simulink model "OT_Test"  (Simulink 8.1)
settings: Solver=ode45  StartTime=0.0  StopTime=100  RelTol=1e-3
values from neighbouring files (symbols this model uses):
  KD1 = x(3)    [FA_FACTS.m]
  KI1 = x(2)    [FA_FACTS.m]
  KP1 = x(1)    [FA_FACTS.m]
  N1 = x(4)    [FA_FACTS.m]
libraries: simulink x1
settings Model: Creator=RS Debdeep Saha  LastModifiedBy=RS Debdeep Saha
settings SolverCC: ZeroCrossControl=DisableAll
settings DataIOCC: SignalLoggingSaveFormat=Dataset
settings OptimizationCC: ExpressionDepthLimit=128
settings DebuggingCC: FcnCallInpInsideContextMsg=EnableAllAsError
settings GRTTargetCC: CombineOutputUpdateFcns=on  GRTInterface=off

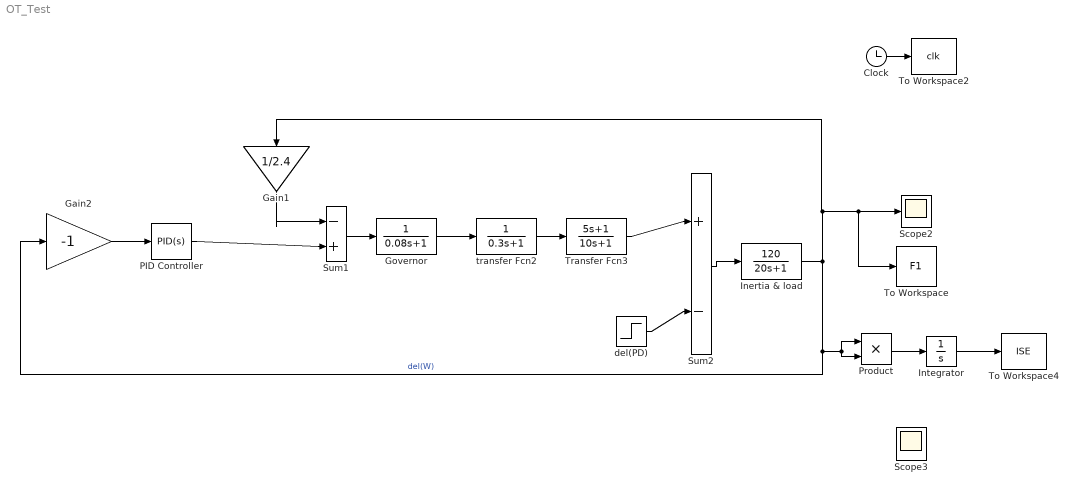
== system OT_Test ==
  Clock : Clock
  Gain1 : Gain  Gain=1/2.4
  Gain2 : Gain  Gain=-1
  Governor : TransferFcn  Denominator=[0.08 1]
  Inertia & load : TransferFcn  Numerator=[120]  Denominator=[20 1]
  Integrator : Integrator
  PID Controller : simulink/Continuous/PID Controller  Controller=PID  TimeDomain=Continuous-time  SampleTime=1  IntegratorMethod=Forward Euler  FilterMethod=Forward Euler  Form=Parallel  P=KP1  I=KI1  D=KD1  N=N1  InitialConditionSource=internal  InitialConditionForIntegrator=0  InitialConditionForFilter=0  ExternalReset=none  LimitOutput=off  UpperSaturationLimit=inf  LowerSaturationLimit=-inf  LinearizeAsGain=on  AntiWindupMode=none  Kb=1  TrackingMode=off  Kt=1  PParamMin=[]  PParamMax=[]  IParamMin=[]  IParamMax=[]  DParamMin=[]  DParamMax=[]  NParamMin=[]  NParamMax=[]  KbParamMin=[]  KbParamMax=[]  KtParamMin=[]  KtParamMax=[]  POutMin=[]  POutMax=[]  IOutMin=[]  IOutMax=[]  DOutMin=[]  DOutMax=[]  NOutMin=[]  NOutMax=[]  KbOutMin=[]  KbOutMax=[]  KtOutMin=[]  KtOutMax=[]  IntegratorOutMin=[]  IntegratorOutMax=[]  FilterOutMin=[]  FilterOutMax=[]  SumOutMin=[]  SumOutMax=[]  SumI1OutMin=[]  SumI1OutMax=[]  SumI2OutMin=[]  SumI2OutMax=[]  SumI3OutMin=[]  SumI3OutMax=[]  SumDOutMin=[]  SumDOutMax=[]  SaturationOutMin=[]  SaturationOutMax=[]  IntegratorContinuousStateAttributes=''  IntegratorStateMustResolveToSignalObject=off  IntegratorRTWStateStorageClass=Auto  FilterContinuousStateAttributes=''  FilterStateMustResolveToSignalObject=off  FilterRTWStateStorageClass=Auto
  Product : Product
  Scope2 : Scope
      settings: SaveName=ScopeData2
  Scope3 : Scope  NumInputPorts=2
      settings: YMin=-5~-5  YMax=5~5
  Sum1 : Sum  Inputs=|-+|
  Sum2 : Sum  Inputs=|+|-
  To Workspace : ToWorkspace  VariableName=F1  SampleTime=-1
  To Workspace2 : ToWorkspace  VariableName=clk  SampleTime=-1
  To Workspace4 : ToWorkspace  VariableName=ISE  SampleTime=-1
  Transfer Fcn3 : TransferFcn  Numerator=[5 1]  Denominator=[10 1]
  del(PD) : Step  Time=0  After=0.02  SampleTime=0
  transfer Fcn2 : TransferFcn  Denominator=[0.3 1]
  wires:
  PID Controller/1 -> Sum1/2
  Gain1/1 -> Sum1/1
  Sum1/1 -> Governor/1
  del(PD)/1 -> Sum2/2
  Sum2/1 -> Inertia & load/1
  Inertia & load/1 -> To Workspace/1, Scope2/1, Gain1/1, Product/2, Product/1, Gain2/1  "del(W)"
  Transfer Fcn3/1 -> Sum2/1
  transfer Fcn2/1 -> Transfer Fcn3/1
  Governor/1 -> transfer Fcn2/1
  Clock/1 -> To Workspace2/1
  Product/1 -> Integrator/1
  Integrator/1 -> To Workspace4/1
  Gain2/1 -> PID Controller/1
